simulink model "Modello_Dirigibile_Quota"  (R2013a)
settings: Solver=ode45  StartTime=0.0  StopTime=30  RelTol=1e-5
settings Model: Creator=Pera  LastModifiedBy=Pera

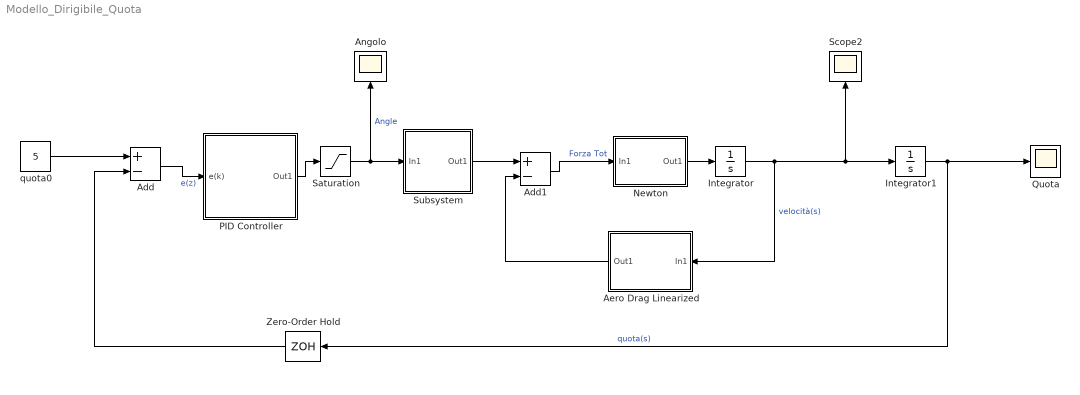
== system Modello_Dirigibile_Quota ==
  Add : Sum  Inputs=+-
  Add1 : Sum  Inputs=+-
  Aero Drag Linearized : Subsystem  mask{rho=1.225, radius=0.5, cd=0.5}
      mask prompts: rho "density"; cd "drag coeff"
      mask init:
      | s1=['rho= ',num2str(rho)];
      | s2=['radius= ',num2str(radius)];
      | s3=['cd= ',num2str(cd)];
      | s=strvcat(s1,s2,s3);  %sto concatenando verticalmente
      mask Display: disp(s)
  Angolo : Scope
      settings: MaxDataPoints=10000
  Integrator : Integrator
  Integrator1 : Integrator
  Newton : Subsystem  mask{m=1}
      mask prompts: m "mass [kg]"
      mask init:
      | s=['mass= ',num2str(m),' [kg]'];
      mask Display: disp(s)
  PID Controller : Subsystem  mask{Ts=0.2, kp=1.5, ki=0.2, kd=2}
      mask prompts: Ts "Sample Time"; kp "Guadagno Proporzionale"; ki "Guadagno Integrativo"; kd "Guadagno Derivativo"
      mask init:
      | s1=['kp= ',num2str(kp)];
      | s2=['ki= ',num2str(ki)];
      | s3=['kd= ',num2str(kd)];
      | s=strvcat(s1,s2,s3);  %sto concatenando verticalmente
      mask Display:
      | disp(s)
      | 
      | image('logo_skyward')
  Quota : Scope
  Saturation : Saturate  UpperLimit=0.7  LowerLimit=-0.7
  Scope2 : Scope
      settings: SaveName=ScopeData2  MaxDataPoints=10000
  Subsystem : Subsystem  mask{T=0.6}
      mask prompts: T "Spinta"
      mask init:
      | s=['T= ',num2str(T),' [N]'];
      mask Display: disp(s)
  Zero-Order Hold : ZeroOrderHold  SampleTime=0.2
  quota0 : Constant  Value=5
  wires:
  Add/1 -> PID Controller/1(e(k))  "e(z)"
  Integrator/1 -> Aero Drag Linearized/1(In1), Integrator1/1, Scope2/1  "velocità(s)"
  Integrator1/1 -> Quota/1, Zero-Order Hold/1  "quota(s)"
  PID Controller/1(Out1) -> Saturation/1
  Zero-Order Hold/1 -> Add/2
  Saturation/1 -> Subsystem/1(In1), Angolo/1  "Angle"
  Add1/1 -> Newton/1(In1)  "Forza Tot"
  Newton/1(Out1) -> Integrator/1
  Aero Drag Linearized/1(Out1) -> Add1/2
  quota0/1 -> Add/1
  Subsystem/1(Out1) -> Add1/1

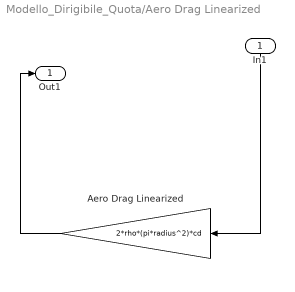
== system Modello_Dirigibile_Quota/Aero Drag Linearized ==
  In1 : Inport
  Aero Drag Linearized : Gain  Gain=2*rho*(pi*radius^2)*cd
  Out1 : Outport
  wires:
  In1/1 -> Aero Drag Linearized/1
  Aero Drag Linearized/1 -> Out1/1

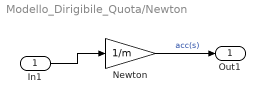
== system Modello_Dirigibile_Quota/Newton ==
  In1 : Inport
  Newton : Gain  Gain=1/m
  Out1 : Outport
  wires:
  In1/1 -> Newton/1
  Newton/1 -> Out1/1  "acc(s)"

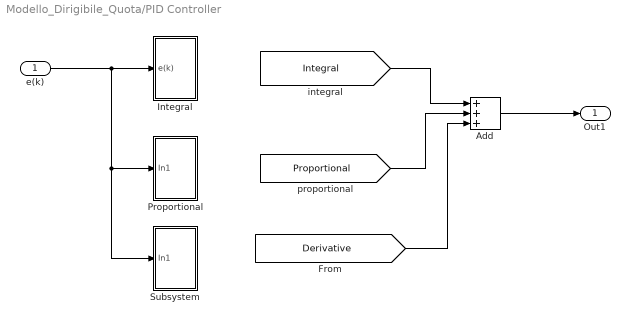
== system Modello_Dirigibile_Quota/PID Controller ==
  e(k) : Inport
  Add : Sum  Inputs=+++
  Integral : Subsystem
  Proportional : Subsystem
  Subsystem : Subsystem
  Out1 : Outport
  wires:
  [Integral] -> Add/1
  Add/1 -> Out1/1
  [Proportional] -> Add/2
  e(k)/1 -> Subsystem/1(In1), Proportional/1(In1), Integral/1(e(k))
  [Derivative] -> Add/3

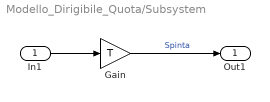
== system Modello_Dirigibile_Quota/Subsystem ==
  In1 : Inport
  Gain : Gain  Gain=T
  Out1 : Outport
  wires:
  Gain/1 -> Out1/1  "Spinta"
  In1/1 -> Gain/1

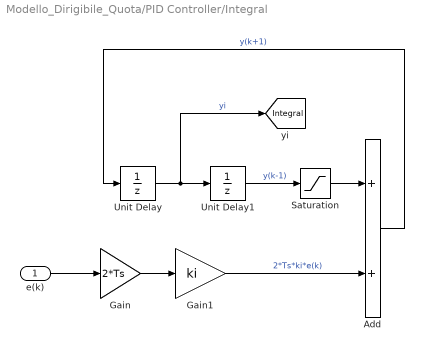
== system Modello_Dirigibile_Quota/PID Controller/Integral ==
  e(k) : Inport
  Add : Sum
  Gain : Gain  Gain=2*Ts
  Gain1 : Gain  Gain=ki
  Saturation : Saturate  UpperLimit=1  LowerLimit=-1
      settings: AttributesFormatString=|
      | %<LowerLimit>
      | %<UpperLimit>
  Unit Delay : UnitDelay  SampleTime=Ts
  Unit Delay1 : UnitDelay  SampleTime=Ts
  tag scope: Integral=global
  wires:
  Gain1/1 -> Add/2  "2*Ts*ki*e(k)"
  Unit Delay/1 -> [Integral], Unit Delay1/1  "yi"
  Gain/1 -> Gain1/1
  Saturation/1 -> Add/1
  Unit Delay1/1 -> Saturation/1  "y(k-1)"
  e(k)/1 -> Gain/1
  Add/1 -> Unit Delay/1  "y(k+1)"

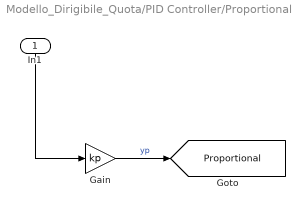
== system Modello_Dirigibile_Quota/PID Controller/Proportional ==
  In1 : Inport
  Gain : Gain  Gain=kp
  tag scope: Proportional=global
  wires:
  Gain/1 -> [Proportional]  "yp"
  In1/1 -> Gain/1

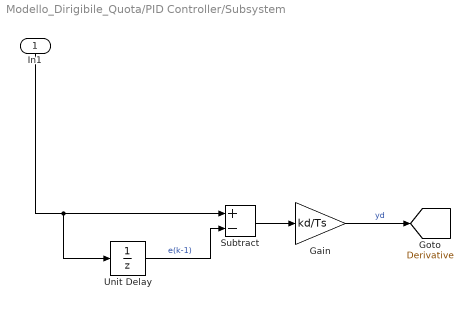
== system Modello_Dirigibile_Quota/PID Controller/Subsystem ==
  In1 : Inport
  Gain : Gain  Gain=kd/Ts
  Subtract : Sum  Inputs=+-
  Unit Delay : UnitDelay  SampleTime=-1
  tag scope: Derivative=global
  wires:
  Unit Delay/1 -> Subtract/2  "e(k-1)"
  Gain/1 -> [Derivative]  "yd"
  Subtract/1 -> Gain/1
  In1/1 -> Unit Delay/1, Subtract/1
